simulink model "can8auto"  (R2018a)
settings: Solver=VariableStepAuto  StartTime=0.0  StopTime=5000  RelTol=1e-3
libraries: commcrc2 x20, simulink x20, simulink_extras x5, dspswit3 x5
(part 1 of 7)
settings Model: Creator=eugi  LastModifiedBy=Davide
settings DebuggingCC: UnderspecifiedInitializationDetection=Classic  LibraryContextMissingDiagnostic=warning
settings SFSimCC: SimUseLocalCustomCode=on
settings RTWCC: RTWUseLocalCustomCode=on

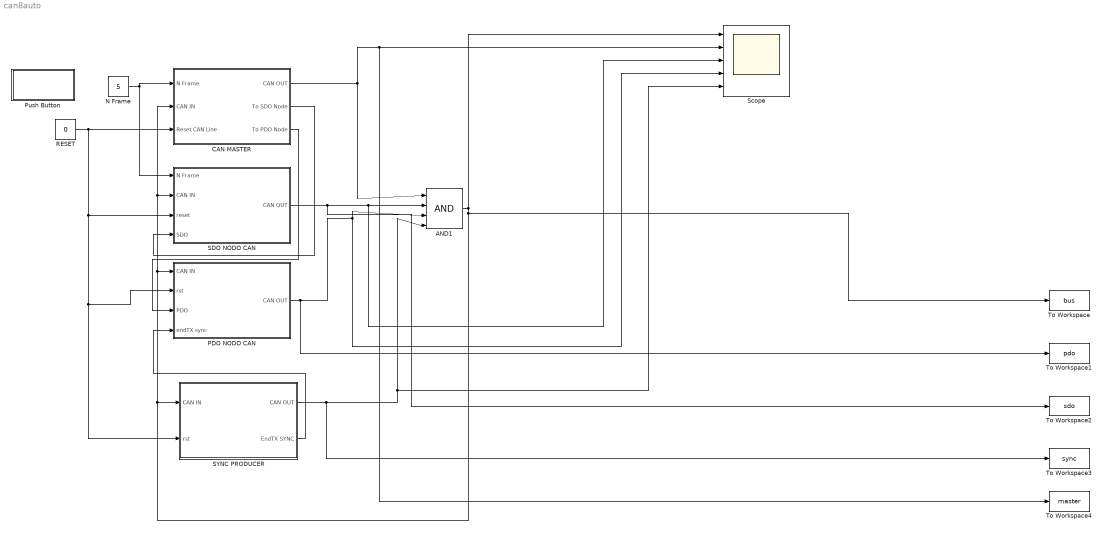
== system can8auto ==
  AND1 : Logic  Inputs=4  IconShape=distinctive  AllPortsSameDT=off  OutDataTypeStr=boolean
  CAN MASTER : Subsystem
  N Frame : Constant  Value=5
  "PDO NODO CAN " : Subsystem
  Push Button : Subsystem  DialogController=hmiCreateDDGDialog  IsWebBlock=on  mask(MWDashboardBlock){webBlockId=d599c260-cdec-44c3-9960-ce2c37887e91, webBlockType=pushbutton, ShowInLibBrowser=on, ShowInitialText=on, HMISrcModelName=can8auto}
      mask prompts: webBlockId "WebBlock Id"; webBlockType "WebBlock Type"; HMISrcModelName "Source Model"
      mask help: Set a value of a tunable parameter or variable by selecting and holding the button. When the push button is not selected, the value is set back to the default value.
      mask Help: helpview([docroot '/mapfiles/simulink.map'], 'hmi_pushbutton')
      mask Display:
      | if strcmp(get_param(bdroot(gcb),'BlockDiagramType'),'library')
      |  image([(matlabroot) '/toolbox/simulink/hmi/icons/PushButton.png'])
      | end
  RESET : Constant  Value=0
  SDO NODO CAN : Subsystem
  SYNC PRODUCER : Subsystem
  Scope : Scope  NumInputPorts=5
  To Workspace : ToWorkspace  VariableName=bus  SaveFormat=Timeseries  SampleTime=-1
  To Workspace1 : ToWorkspace  VariableName=pdo  SaveFormat=Timeseries  SampleTime=-1
  To Workspace2 : ToWorkspace  VariableName=sdo  SaveFormat=Timeseries  SampleTime=-1
  To Workspace3 : ToWorkspace  VariableName=sync  SaveFormat=Timeseries  SampleTime=-1
  To Workspace4 : ToWorkspace  VariableName=master  SaveFormat=Timeseries  SampleTime=-1
  wires:
  N Frame/1 -> SDO NODO CAN/1(N Frame), CAN MASTER/1(N Frame)
  RESET/1 -> CAN MASTER/3(Reset CAN Line), SDO NODO CAN/3(reset), "PDO NODO CAN "/2(rst), SYNC PRODUCER/2(rst)
  CAN MASTER/2(To SDO Node) -> SDO NODO CAN/4(SDO)
  CAN MASTER/3(To PDO Node) -> "PDO NODO CAN "/3(PDO)
  SYNC PRODUCER/2(EndTX SYNC) -> "PDO NODO CAN "/4(endTX sync)
  CAN MASTER/1(CAN OUT) -> AND1/1, To Workspace4/1, Scope/2
  SYNC PRODUCER/1(CAN OUT) -> To Workspace3/1, AND1/4, Scope/5
  SDO NODO CAN/1(CAN OUT) -> To Workspace2/1, Scope/3, AND1/2
  AND1/1 -> Scope/1, To Workspace/1, SYNC PRODUCER/1(CAN IN), SDO NODO CAN/2(CAN IN), CAN MASTER/2(CAN IN), "PDO NODO CAN "/1(CAN IN)
  "PDO NODO CAN "/1(CAN OUT) -> To Workspace1/1, Scope/4, AND1/3

== system can8auto/CAN MASTER ==
  N Frame : Inport
  CAN IN : Inport  Port=2
  Reset CAN Line : Inport  Port=3
  CAN NODE : Subsystem
  Chart : Stateflow chart  TreatAsAtomicUnit=on
  Clock : simulink_extras/Flip Flops/Clock  period=0.000001
  Constant : Constant
  Counter : dspswit3/Counter  Direction=Up  CountEvent=Rising edge  CounterSize=User defined  MaxCount=255  InitialCount=0  Output=Count and Hit  HitValue=32  ResetInput=on  SamplesPerFrame=1  Ts=1  CntDtype=double  HitDtype=Logical
  Counter1 : dspswit3/Counter  Direction=Up  CountEvent=Rising edge  CounterSize=User defined  MaxCount=255  InitialCount=0  Output=Count and Hit  HitValue=32  ResetInput=on  SamplesPerFrame=1  Ts=1  CntDtype=double  HitDtype=Logical
  Equal : RelationalOperator  Operator=~=  OutDataTypeStr=boolean  RndMeth=Simplest
  MATLAB Function : MATLAB Function  TreatAsAtomicUnit=on
  MATLAB Function1 : MATLAB Function  TreatAsAtomicUnit=on
  Master : Stateflow chart  TreatAsAtomicUnit=on
  Memory1 : Memory  InitialCondition=1
  Memory2 : Memory  InheritSampleTime=on
  Memory3 : Memory
  Sensing : Subsystem
  Sum : Sum  Inputs=|++
  XOR : Logic  Operator=XOR  IconShape=distinctive  AllPortsSameDT=off  OutDataTypeStr=boolean
  CAN OUT : Outport
  To SDO Node : Outport  Port=2
  To PDO Node : Outport  Port=3
  wires:
  Chart/1(state) -> Sensing/3(Enable CS), MATLAB Function/3(state)
  Clock/1 -> MATLAB Function/Trigger, Sensing/2(clock)
  Sensing/1(Free) -> Chart/1(Free)
  CAN IN/1 -> XOR/1, Sensing/1(BusState)
  XOR/1 -> Memory3/1
  CAN NODE/1(Frame Message) -> MATLAB Function/1(parallel)
  Memory1/1 -> MATLAB Function/2(current_index)
  MATLAB Function/2(next_index) -> Memory1/1
  MATLAB Function/1(serial) -> MATLAB Function1/1(u)
  MATLAB Function/3(endTX) -> Memory2/1
  MATLAB Function1/1(y) -> CAN OUT/1, XOR/2
  Memory3/1 -> Chart/2(Error)
  Memory2/1 -> Counter1/1, CAN NODE/1(End TX), Counter/1, Master/2(EndTX), Chart/4(EndTX)
  Master/3(sigOut) -> CAN NODE/2(TX Kind)
  Reset CAN Line/1 -> Counter/2, Master/1(rst)
  Master/1(SDO) -> To SDO Node/1
  Master/2(PDO) -> To PDO Node/1
  Counter/1 -> Master/3(totalTX)
  Counter1/1 -> Equal/2
  Equal/1 -> Chart/3(Frame)
  Constant/1 -> Sum/2
  N Frame/1 -> Sum/1
  Sum/1 -> Equal/1

== system can8auto/PDO NODO CAN  ==
  CAN IN : Inport
  rst : Inport  Port=2
  PDO : Inport  Port=3
  endTX sync : Inport  Port=4
  AND : Logic  IconShape=distinctive  AllPortsSameDT=off  OutDataTypeStr=boolean
  CAN NODE : Subsystem
  Chart : Stateflow chart  TreatAsAtomicUnit=on
  Clock : simulink_extras/Flip Flops/Clock  period=0.000001
  Counter of Sync Messages : Subsystem
  Delay : Delay  DelayLength=3
  Delay1 : Delay
  MATLAB Function : MATLAB Function  TreatAsAtomicUnit=on
  MATLAB Function1 : MATLAB Function  TreatAsAtomicUnit=on
  MATLAB Function2 : MATLAB Function  TreatAsAtomicUnit=on
  Memory1 : Memory  InitialCondition=1
  Memory2 : Memory  InheritSampleTime=on
  Memory3 : Memory
  NOT : Logic  Operator=NOT  IconShape=distinctive  AllPortsSameDT=off  OutDataTypeStr=boolean
  OR : Logic  Operator=OR  IconShape=distinctive  AllPortsSameDT=off  OutDataTypeStr=boolean
  Rate Transition : RateTransition
  Sensing : Subsystem
  SlavePDO : Stateflow chart  TreatAsAtomicUnit=on
  Start on push : Subsystem
  XOR : Logic  Operator=XOR  IconShape=distinctive  AllPortsSameDT=off  OutDataTypeStr=boolean
  CAN OUT : Outport
  wires:
  Chart/1(state) -> Sensing/3(Enable CS), MATLAB Function/3(state)
  Clock/1 -> AND/2, Start on push/1(New TX), MATLAB Function/Trigger, Sensing/2(clock)
  Sensing/1(Free) -> Chart/1(Free)
  CAN IN/1 -> XOR/1, Sensing/1(BusState)
  XOR/1 -> Memory3/1
  CAN NODE/1(Frame Message) -> MATLAB Function/1(parallel)
  Memory1/1 -> MATLAB Function/2(current_index)
  MATLAB Function/2(next_index) -> Memory1/1
  MATLAB Function/1(serial) -> MATLAB Function1/1(u)
  MATLAB Function/3(endTX) -> Memory2/1
  MATLAB Function1/1(y) -> CAN OUT/1, XOR/2
  Memory2/1 -> OR/2, Counter of Sync Messages/2(Down), SlavePDO/3(EndTX), Chart/4(EndTX)
  Memory3/1 -> Chart/2(Error)
  SlavePDO/1(mode) -> NOT/1, CAN NODE/2("Tx kind "), Chart/6(mode)
  rst/1 -> SlavePDO/1(rst)
  PDO/1 -> SlavePDO/2(PDO)
  endTX sync/1 -> Counter of Sync Messages/1(Up)
  Counter of Sync Messages/1(NFrame) -> Rate Transition/1
  Rate Transition/1 -> Chart/3(trigger)
  AND/1 -> OR/1
  NOT/1 -> AND/1
  Start on push/1(Out1) -> Delay/1
  Delay/1 -> Chart/5(NewTX)
  OR/1 -> Delay1/1
  Delay1/1 -> CAN NODE/1(Transmission Ready)

== system can8auto/Push Button ==

== system can8auto/SDO NODO CAN ==
  N Frame : Inport
  CAN IN : Inport  Port=2
  reset : Inport  Port=3
  SDO : Inport  Port=4
  CAN NODE : Subsystem
  Chart : Stateflow chart  TreatAsAtomicUnit=on
  Clock : simulink_extras/Flip Flops/Clock  period=0.000001
  Constant : Constant
  Counter : dspswit3/Counter  Direction=Up  CountEvent=Rising edge  CounterSize=User defined  MaxCount=255  InitialCount=0  Output=Count and Hit  HitValue=32  ResetInput=on  SamplesPerFrame=1  Ts=1  CntDtype=double  HitDtype=Logical
  Counter1 : dspswit3/Counter  Direction=Up  CountEvent=Rising edge  CounterSize=User defined  MaxCount=255  InitialCount=0  Output=Count and Hit  HitValue=32  ResetInput=on  SamplesPerFrame=1  Ts=1  CntDtype=double  HitDtype=Logical
  Equal : RelationalOperator  Operator=~=  OutDataTypeStr=boolean  RndMeth=Simplest
  MATLAB Function : MATLAB Function  TreatAsAtomicUnit=on
  MATLAB Function1 : MATLAB Function  TreatAsAtomicUnit=on
  Memory1 : Memory  InitialCondition=1
  Memory2 : Memory  InheritSampleTime=on
  Memory3 : Memory
  Sensing : Subsystem
  SlaveSDO : Stateflow chart  TreatAsAtomicUnit=on
  Sum : Sum  Inputs=|++
  XOR : Logic  Operator=XOR  IconShape=distinctive  AllPortsSameDT=off  OutDataTypeStr=boolean
  CAN OUT : Outport
  wires:
  Chart/1(state) -> Sensing/3(Enable CS), MATLAB Function/3(state)
  Clock/1 -> MATLAB Function/Trigger, Sensing/2(clock)
  Sensing/1(Free) -> Chart/1(Free)
  CAN IN/1 -> XOR/1, Sensing/1(BusState)
  XOR/1 -> Memory3/1
  CAN NODE/1(Frame Message) -> MATLAB Function/1(parallel)
  Memory1/1 -> MATLAB Function/2(current_index)
  MATLAB Function/2(next_index) -> Memory1/1
  MATLAB Function/1(serial) -> MATLAB Function1/1(u)
  MATLAB Function/3(endTX) -> Memory2/1
  MATLAB Function1/1(y) -> CAN OUT/1, XOR/2
  Memory3/1 -> Chart/2(Error)
  reset/1 -> Counter/2, SlaveSDO/1(rst)
  SDO/1 -> SlaveSDO/2(SDO)
  SlaveSDO/1(mode) -> CAN NODE/2(Frame kind)
  Counter/1 -> SlaveSDO/3(TotTX)
  Equal/1 -> Chart/3(Frame)
  Sum/1 -> Equal/1
  N Frame/1 -> Sum/1
  Counter1/1 -> Equal/2
  Constant/1 -> Sum/2
  Memory2/1 -> Counter1/1, Counter/1, SlaveSDO/4(EndTX), CAN NODE/1(End TX), Chart/4(EndTX)

== system can8auto/SYNC PRODUCER ==
  CAN IN : Inport
  rst : Inport  Port=2
  AND : Logic  Inputs=3  IconShape=distinctive  AllPortsSameDT=off  OutDataTypeStr=boolean
  CAN NODE : Subsystem
  Chart : Stateflow chart  TreatAsAtomicUnit=on
  Chart1 : Stateflow chart  TreatAsAtomicUnit=on
  Clock : simulink_extras/Flip Flops/Clock  period=0.000001
  Clock1 : simulink_extras/Flip Flops/Clock  period=0.000002
  Counter1 : dspswit3/Counter  Direction=Up  CountEvent=Rising edge  CounterSize=User defined  MaxCount=256  InitialCount=0  Output=Count and Hit  HitValue=256  ResetInput=on  SamplesPerFrame=1  Ts=1  CntDtype=double  HitDtype=Logical
  Delay : Delay  DelayLength=3
  Display2 : Display
  MATLAB Function : MATLAB Function  TreatAsAtomicUnit=on
  Memory : Memory
  Memory1 : Memory  InitialCondition=1
  Memory2 : Memory  InheritSampleTime=on
  Memory3 : Memory
  Memory4 : Memory  InheritSampleTime=on
  NOT : Logic  Operator=NOT  IconShape=distinctive  AllPortsSameDT=off  OutDataTypeStr=boolean
  OR : Logic  Operator=OR  IconShape=distinctive  AllPortsSameDT=off  OutDataTypeStr=boolean
  P/S converter : MATLAB Function  TreatAsAtomicUnit=on
  Rate Transition : RateTransition
  Sensing : Subsystem
  Start on push : Subsystem
  XOR : Logic  Operator=XOR  IconShape=distinctive  AllPortsSameDT=off  OutDataTypeStr=boolean
  double to boolean : MATLAB Function  TreatAsAtomicUnit=on
  CAN OUT : Outport
  EndTX SYNC : Outport  Port=2
  wires:
  Chart/1(state) -> Sensing/3(Enable CS), Memory4/1, P/S converter/3(state)
  Sensing/1(Free) -> Chart/1(Free)
  CAN IN/1 -> XOR/1, Sensing/1(BusState)
  XOR/1 -> Memory3/1
  CAN NODE/1(Frame Message) -> P/S converter/1(parallel)
  Memory1/1 -> P/S converter/2(current_index)
  P/S converter/2(next_index) -> Memory1/1
  P/S converter/1(serial) -> double to boolean/1(u)
  P/S converter/3(endTX) -> Memory2/1
  double to boolean/1(y) -> CAN OUT/1, XOR/2
  Memory2/1 -> OR/2, Chart1/1(EndTX), EndTX SYNC/1, Chart/3(EndTX)
  Memory3/1 -> Chart/2(Error)
  rst/1 -> Chart1/2(rst), OR/1
  Chart1/1(mode) -> Chart/6(mode), MATLAB Function/1(u), CAN NODE/2(tx kind)
  Clock1/1 -> AND/1
  AND/1 -> Counter1/1
  Memory/1 -> Rate Transition/1
  Rate Transition/1 -> AND/2
  Counter1/1 -> Display2/1
  Clock/1 -> Start on push/1(New TX), CAN NODE/1(Transmission Ready), P/S converter/Trigger, Sensing/2(clock)
  Start on push/1(Out1) -> Delay/1
  MATLAB Function/1(y) -> Memory/1
  Counter1/2 -> Chart/5(tempo)
  NOT/1 -> AND/3
  Memory4/1 -> NOT/1
  OR/1 -> Counter1/2
  Delay/1 -> Chart/4(enableTX)

== system can8auto/CAN MASTER/CAN NODE ==
  note: DA INSERIRE L'ID DEL NODO
      | (Node ID) & L'INDIRIZZO
      | RICEVITORE DI UN NMT NODE
      | (Address Node)
  note: TRANSMISSION TRIGGER
  note: MESSAGE CONIG
  End TX : Inport
  TX Kind : Inport  Port=2
  "Address Node " : Constant  Value=[0,0,0,0,0,0,0,0,0,0,0]  VectorParams1D=off
  Bootup Frame generator : Subsystem
  Complex to Real-Imag : ComplexToRealImag  Output=Real
  Frame MUX : Subsystem
  Length : Constant  Value=4  VectorParams1D=off
  Mode : Constant  VectorParams1D=off
  NMT Frame generator : Subsystem
  Node ID : Constant  Value=[0,0,1,0,0,0,0,1,1,1,1]  VectorParams1D=off
  PDO Frame Generator : Subsystem
  Radio Button : RadioButtonGroup  WebBlockId=15712  LabelPosition=Hide  SelectedLabel=Bootup Message  ButtonGroupName=Message
      settings: Values={{'Bootup Message', 'NMT Message', 'SDO Message', 'PDO Message', 'SYNC Message'}, [0 1 2 3 4]}
  Radio Button1 : RadioButtonGroup  WebBlockId=15713  LabelPosition=Hide  SelectedLabel=WriteClent  ButtonGroupName=SDO request
      settings: Values={{'ReadClient', 'WriteClent', 'ReadServer', 'WriteServer'}, [0 1 2 3]}
  Radio Button2 : RadioButtonGroup  WebBlockId=15714  LabelPosition=Hide  SelectedLabel=4 Byte  ButtonGroupName=PDO Length
      settings: Values={{'2 Byte', '4 Byte', '8 Byte'}, [2 4 8]}
  SDO Frame generator : Subsystem
  SYNC Frame Generator : Subsystem
  Triggered Subsystem1 : Subsystem  TreatAsAtomicUnit=on
  Frame Message : Outport
  wires:
  Complex to Real-Imag/1 -> Frame Message/1
  Frame MUX/1(Frame to Send) -> Triggered Subsystem1/1(In1)
  "Address Node "/1 -> NMT Frame generator/1(Address node)
  TX Kind/1 -> Frame MUX/1(Frame Kind)
  NMT Frame generator/2(" Size") -> Frame MUX/5(Size NMT)
  SYNC Frame Generator/2(" Size") -> Frame MUX/11(Size SYNC)
  Mode/1 -> SDO Frame generator/2(Mode)
  Length/1 -> PDO Frame Generator/2(Data Length)
  Bootup Frame generator/2(" Size") -> Frame MUX/3(Size Bootload)
  SDO Frame generator/2(" Size") -> Frame MUX/7(Size SDO)
  Node ID/1 -> Bootup Frame generator/1(ID of the Node), PDO Frame Generator/1(CAN ID), SDO Frame generator/1(CAN ID of the Node)
  NMT Frame generator/1(NMT Frame) -> Frame MUX/4(NMT Frame)
  PDO Frame Generator/2(" Size") -> Frame MUX/9(Size PDO)
  SDO Frame generator/1(SDO Frame) -> Frame MUX/6(SDO Frame)
  SYNC Frame Generator/1(SYNC Frame) -> Frame MUX/10(SYNC Frame)
  Bootup Frame generator/1(Bootload Frame) -> Frame MUX/2(Bootload Frame)
  PDO Frame Generator/1(PDO Frame) -> Frame MUX/8(PDO Frame)
  Triggered Subsystem1/1(Out1) -> Complex to Real-Imag/1
  End TX/1 -> Triggered Subsystem1/Trigger

== system can8auto/CAN MASTER/Sensing ==
  BusState : Inport
  clock : Inport  Port=2
  Enable CS : Inport  Port=3
  AND : Logic  IconShape=distinctive  AllPortsSameDT=off  OutDataTypeStr=boolean
  Data Store Memory : DataStoreMemory  ReadBeforeWriteMsg=warning  WriteAfterWriteMsg=warning  WriteAfterReadMsg=warning  ShowAdditionalParam=off
  Data Store Read : DataStoreRead
  Data Store Write : DataStoreWrite
  MATLAB Function : MATLAB Function  TreatAsAtomicUnit=on
  Memory : Memory
  NOT : Logic  Operator=NOT  IconShape=distinctive  AllPortsSameDT=off  OutDataTypeStr=boolean
  Free : Outport
  wires:
  Memory/1 -> Free/1
  Enable CS/1 -> AND/1
  AND/1 -> NOT/1
  clock/1 -> AND/2
  NOT/1 -> MATLAB Function/Trigger, MATLAB Function/2(clock)
  MATLAB Function/2(count) -> Data Store Write/1
  Data Store Read/1 -> MATLAB Function/3("count ")
  MATLAB Function/1(free) -> Memory/1
  BusState/1 -> MATLAB Function/1(BusState)

== system can8auto/PDO NODO CAN /CAN NODE ==
  note: DA INSERIRE L'ID DEL NODO
      | (Node ID) & L'INDIRIZZO
      | RICEVITORE DI UN NMT NODE
      | (Address Node)
  note: TRANSMISSION TRIGGER
  note: MESSAGE CONIG
  Transmission Ready : Inport
  "Tx kind " : Inport  Port=2
  "Address Node " : Constant  Value=[0,0,0,0,0,0,0,0,0,0,0]  VectorParams1D=off
  Bootup Frame generator : Subsystem
  Complex to Real-Imag : ComplexToRealImag  Output=Real
  Frame MUX : Subsystem
  Length : Constant  Value=4  VectorParams1D=off
  Mode : Constant  VectorParams1D=off
  NMT Frame generator : Subsystem
  Node ID : Constant  Value=[0,0,1,1,0,0,0,0,1,0,1]  VectorParams1D=off
  PDO Frame Generator : Subsystem
  Radio Button : RadioButtonGroup  WebBlockId=13844  LabelPosition=Hide  SelectedLabel=Bootup Message  ButtonGroupName=Message
      settings: Values={{'Bootup Message', 'NMT Message', 'SDO Message', 'PDO Message', 'SYNC Message'}, [0 1 2 3 4]}
  Radio Button1 : RadioButtonGroup  WebBlockId=13845  LabelPosition=Hide  SelectedLabel=WriteClent  ButtonGroupName=SDO request
      settings: Values={{'ReadClient', 'WriteClent', 'ReadServer', 'WriteServer'}, [0 1 2 3]}
  Radio Button2 : RadioButtonGroup  WebBlockId=13846  LabelPosition=Hide  SelectedLabel=4 Byte  ButtonGroupName=PDO Length
      settings: Values={{'2 Byte', '4 Byte', '8 Byte'}, [2 4 8]}
  SDO Frame generator : Subsystem
  SYNC Frame Generator : Subsystem
  Triggered Subsystem1 : Subsystem  TreatAsAtomicUnit=on
  Frame Message : Outport
  wires:
  Transmission Ready/1 -> Triggered Subsystem1/Trigger
  Complex to Real-Imag/1 -> Frame Message/1
  Frame MUX/1(Frame to Send) -> Triggered Subsystem1/1(In1)
  "Address Node "/1 -> NMT Frame generator/1(Address node)
  "Tx kind "/1 -> Frame MUX/1(Frame Kind)
  NMT Frame generator/2(" Size") -> Frame MUX/5(Size NMT)
  SYNC Frame Generator/2(" Size") -> Frame MUX/11(Size SYNC)
  Mode/1 -> SDO Frame generator/2(Mode)
  Length/1 -> PDO Frame Generator/2(Data Length)
  Bootup Frame generator/2(" Size") -> Frame MUX/3(Size Bootload)
  SDO Frame generator/2(" Size") -> Frame MUX/7(Size SDO)
  Node ID/1 -> Bootup Frame generator/1(ID of the Node), PDO Frame Generator/1(CAN ID), SDO Frame generator/1(CAN ID of the Node)
  NMT Frame generator/1(NMT Frame) -> Frame MUX/4(NMT Frame)
  PDO Frame Generator/2(" Size") -> Frame MUX/9(Size PDO)
  SDO Frame generator/1(SDO Frame) -> Frame MUX/6(SDO Frame)
  SYNC Frame Generator/1(SYNC Frame) -> Frame MUX/10(SYNC Frame)
  Bootup Frame generator/1(Bootload Frame) -> Frame MUX/2(Bootload Frame)
  PDO Frame Generator/1(PDO Frame) -> Frame MUX/8(PDO Frame)
  Triggered Subsystem1/1(Out1) -> Complex to Real-Imag/1

== system can8auto/PDO NODO CAN /Counter of Sync Messages ==
  Up : Inport
  Down : Inport  Port=2
  ADDER : MATLAB Function  TreatAsAtomicUnit=on
  Memory : Memory
  OR : Logic  Operator=OR  IconShape=distinctive  AllPortsSameDT=off  OutDataTypeStr=boolean
  NFrame : Outport
  wires:
  Up/1 -> ADDER/1(up), OR/2
  Memory/1 -> ADDER/3(counter), NFrame/1
  Down/1 -> ADDER/2(down), OR/1
  OR/1 -> ADDER/Trigger
  ADDER/1(val) -> Memory/1

== system can8auto/PDO NODO CAN /Sensing ==
  BusState : Inport
  clock : Inport  Port=2
  Enable CS : Inport  Port=3
  AND : Logic  IconShape=distinctive  AllPortsSameDT=off  OutDataTypeStr=boolean
  Data Store Memory : DataStoreMemory  ReadBeforeWriteMsg=warning  WriteAfterWriteMsg=warning  WriteAfterReadMsg=warning  ShowAdditionalParam=off
  Data Store Read : DataStoreRead
  Data Store Write : DataStoreWrite
  MATLAB Function : MATLAB Function  TreatAsAtomicUnit=on
  Memory : Memory
  NOT : Logic  Operator=NOT  IconShape=distinctive  AllPortsSameDT=off  OutDataTypeStr=boolean
  Free : Outport
  wires:
  Memory/1 -> Free/1
  Enable CS/1 -> AND/1
  AND/1 -> NOT/1
  clock/1 -> AND/2
  NOT/1 -> MATLAB Function/Trigger, MATLAB Function/2(clock)
  MATLAB Function/2(count) -> Data Store Write/1
  Data Store Read/1 -> MATLAB Function/3("count ")
  MATLAB Function/1(free) -> Memory/1
  BusState/1 -> MATLAB Function/1(BusState)

== system can8auto/PDO NODO CAN /Start on push ==
  New TX : Inport
  Constant : Constant
  Start on push : Subsystem  TreatAsAtomicUnit=on
  Out1 : Outport
  wires:
  Start on push/1(Out1) -> Out1/1
  New TX/1 -> Start on push/Trigger
  Constant/1 -> Start on push/1(In1)

== system can8auto/SDO NODO CAN/CAN NODE ==
  note: DA INSERIRE L'ID DEL NODO
      | (Node ID) & L'INDIRIZZO
      | RICEVITORE DI UN NMT NODE
      | (Address Node)
  note: TRANSMISSION TRIGGER
  note: MESSAGE CONIG
  End TX : Inport
  Frame kind : Inport  Port=2
  "Address Node " : Constant  Value=[0,0,0,0,0,0,0,0,0,0,0]  VectorParams1D=off
  Bootup Frame generator : Subsystem
  Complex to Real-Imag : ComplexToRealImag  Output=Real
  Frame MUX : Subsystem
  Length : Constant  Value=4  VectorParams1D=off
  Mode : Constant  VectorParams1D=off
  NMT Frame generator : Subsystem
  Node ID : Constant  Value=[0,0,1,1,0,0,1,0,1,0,1]  VectorParams1D=off
  PDO Frame Generator : Subsystem
  Radio Button : RadioButtonGroup  WebBlockId=16646  LabelPosition=Hide  SelectedLabel=Bootup Message  ButtonGroupName=Message
      settings: Values={{'Bootup Message', 'NMT Message', 'SDO Message', 'PDO Message', 'SYNC Message'}, [0 1 2 3 4]}
  Radio Button1 : RadioButtonGroup  WebBlockId=16647  LabelPosition=Hide  SelectedLabel=WriteClent  ButtonGroupName=SDO request
      settings: Values={{'ReadClient', 'WriteClent', 'ReadServer', 'WriteServer'}, [0 1 2 3]}
  Radio Button2 : RadioButtonGroup  WebBlockId=16648  LabelPosition=Hide  SelectedLabel=4 Byte  ButtonGroupName=PDO Length
      settings: Values={{'2 Byte', '4 Byte', '8 Byte'}, [2 4 8]}
  SDO Frame generator : Subsystem
  SYNC Frame Generator : Subsystem
  Triggered Subsystem1 : Subsystem  TreatAsAtomicUnit=on
  Frame Message : Outport
  wires:
  Complex to Real-Imag/1 -> Frame Message/1
  Frame MUX/1(Frame to Send) -> Triggered Subsystem1/1(In1)
  "Address Node "/1 -> NMT Frame generator/1(Address node)
  Frame kind/1 -> Frame MUX/1(Frame Kind)
  NMT Frame generator/2(" Size") -> Frame MUX/5(Size NMT)
  SYNC Frame Generator/2(" Size") -> Frame MUX/11(Size SYNC)
  Mode/1 -> SDO Frame generator/2(Mode)
  Length/1 -> PDO Frame Generator/2(Data Length)
  Bootup Frame generator/2(" Size") -> Frame MUX/3(Size Bootload)
  SDO Frame generator/2(" Size") -> Frame MUX/7(Size SDO)
  Node ID/1 -> Bootup Frame generator/1(ID of the Node), PDO Frame Generator/1(CAN ID), SDO Frame generator/1(CAN ID of the Node)
  NMT Frame generator/1(NMT Frame) -> Frame MUX/4(NMT Frame)
  PDO Frame Generator/2(" Size") -> Frame MUX/9(Size PDO)
  SDO Frame generator/1(SDO Frame) -> Frame MUX/6(SDO Frame)
  SYNC Frame Generator/1(SYNC Frame) -> Frame MUX/10(SYNC Frame)
  Bootup Frame generator/1(Bootload Frame) -> Frame MUX/2(Bootload Frame)
  PDO Frame Generator/1(PDO Frame) -> Frame MUX/8(PDO Frame)
  Triggered Subsystem1/1(Out1) -> Complex to Real-Imag/1
  End TX/1 -> Triggered Subsystem1/Trigger

== system can8auto/SDO NODO CAN/Sensing ==
  BusState : Inport
  clock : Inport  Port=2
  Enable CS : Inport  Port=3
  AND : Logic  IconShape=distinctive  AllPortsSameDT=off  OutDataTypeStr=boolean
  Data Store Memory : DataStoreMemory  ReadBeforeWriteMsg=warning  WriteAfterWriteMsg=warning  WriteAfterReadMsg=warning  ShowAdditionalParam=off
  Data Store Read : DataStoreRead
  Data Store Write : DataStoreWrite
  MATLAB Function : MATLAB Function  TreatAsAtomicUnit=on
  Memory : Memory
  NOT : Logic  Operator=NOT  IconShape=distinctive  AllPortsSameDT=off  OutDataTypeStr=boolean
  Free : Outport
  wires:
  Memory/1 -> Free/1
  Enable CS/1 -> AND/1
  AND/1 -> NOT/1
  clock/1 -> AND/2
  NOT/1 -> MATLAB Function/Trigger, MATLAB Function/2(clock)
  MATLAB Function/2(count) -> Data Store Write/1
  Data Store Read/1 -> MATLAB Function/3("count ")
  MATLAB Function/1(free) -> Memory/1
  BusState/1 -> MATLAB Function/1(BusState)

== system can8auto/SYNC PRODUCER/CAN NODE ==
  note: DA INSERIRE L'ID DEL NODO
      | (Node ID) & L'INDIRIZZO
      | RICEVITORE DI UN NMT NODE
      | (Address Node)
  note: TRANSMISSION TRIGGER
  note: MESSAGE CONIG
  Transmission Ready : Inport
  tx kind : Inport  Port=2
  "Address Node " : Constant  Value=[0,0,0,0,0,0,0,0,0,0,0]  VectorParams1D=off
  Bootup Frame generator : Subsystem
  Complex to Real-Imag : ComplexToRealImag  Output=Real
  Frame MUX : Subsystem
  Length : Constant  Value=4  VectorParams1D=off
  Mode : Constant  VectorParams1D=off
  NMT Frame generator : Subsystem
  Node ID : Constant  Value=[0,0,1,0,0,0,0,1,1,0,1]  VectorParams1D=off
  PDO Frame Generator : Subsystem
  Radio Button1 : RadioButtonGroup  WebBlockId=17625  LabelPosition=Hide  SelectedLabel=WriteClent  ButtonGroupName=SDO request
      settings: Values={{'ReadClient', 'WriteClent', 'ReadServer', 'WriteServer'}, [0 1 2 3]}
  Radio Button2 : RadioButtonGroup  WebBlockId=17626  LabelPosition=Hide  SelectedLabel=4 Byte  ButtonGroupName=PDO Length
      settings: Values={{'2 Byte', '4 Byte', '8 Byte'}, [2 4 8]}
  SDO Frame generator : Subsystem
  SYNC Frame Generator : Subsystem
  Triggered Subsystem1 : Subsystem  TreatAsAtomicUnit=on
  Frame Message : Outport
  wires:
  Transmission Ready/1 -> Triggered Subsystem1/Trigger
  Complex to Real-Imag/1 -> Frame Message/1
  Frame MUX/1(Frame to Send) -> Triggered Subsystem1/1(In1)
  "Address Node "/1 -> NMT Frame generator/1(Address node)
  tx kind/1 -> Frame MUX/1(Frame Kind)
  NMT Frame generator/2(" Size") -> Frame MUX/5(Size NMT)
  SYNC Frame Generator/2(" Size") -> Frame MUX/11(Size SYNC)
  Mode/1 -> SDO Frame generator/2(Mode)
  Length/1 -> PDO Frame Generator/2(Data Length)
  Bootup Frame generator/2(" Size") -> Frame MUX/3(Size Bootload)
  SDO Frame generator/2(" Size") -> Frame MUX/7(Size SDO)
  Node ID/1 -> Bootup Frame generator/1(ID of the Node), PDO Frame Generator/1(CAN ID), SDO Frame generator/1(CAN ID of the Node)
  NMT Frame generator/1(NMT Frame) -> Frame MUX/4(NMT Frame)
  PDO Frame Generator/2(" Size") -> Frame MUX/9(Size PDO)
  SDO Frame generator/1(SDO Frame) -> Frame MUX/6(SDO Frame)
  SYNC Frame Generator/1(SYNC Frame) -> Frame MUX/10(SYNC Frame)
  Bootup Frame generator/1(Bootload Frame) -> Frame MUX/2(Bootload Frame)
  PDO Frame Generator/1(PDO Frame) -> Frame MUX/8(PDO Frame)
  Triggered Subsystem1/1(Out1) -> Complex to Real-Imag/1

== system can8auto/SYNC PRODUCER/Sensing ==
  BusState : Inport
  clock : Inport  Port=2
  Enable CS : Inport  Port=3
  AND : Logic  IconShape=distinctive  AllPortsSameDT=off  OutDataTypeStr=boolean
  Data Store Memory : DataStoreMemory  ReadBeforeWriteMsg=warning  WriteAfterWriteMsg=warning  WriteAfterReadMsg=warning  ShowAdditionalParam=off
  Data Store Read : DataStoreRead
  Data Store Write : DataStoreWrite
  MATLAB Function : MATLAB Function  TreatAsAtomicUnit=on
  Memory : Memory
  NOT : Logic  Operator=NOT  IconShape=distinctive  AllPortsSameDT=off  OutDataTypeStr=boolean
  Free : Outport
  wires:
  Memory/1 -> Free/1
  Enable CS/1 -> AND/1
  AND/1 -> NOT/1
  clock/1 -> AND/2
  NOT/1 -> MATLAB Function/Trigger, MATLAB Function/2(clock)
  MATLAB Function/2(count) -> Data Store Write/1
  Data Store Read/1 -> MATLAB Function/3("count ")
  MATLAB Function/1(free) -> Memory/1
  BusState/1 -> MATLAB Function/1(BusState)

== system can8auto/SYNC PRODUCER/Start on push ==
  New TX : Inport
  Constant : Constant
  Start on push : Subsystem  TreatAsAtomicUnit=on
  Out1 : Outport
  wires:
  Start on push/1(Out1) -> Out1/1
  New TX/1 -> Start on push/Trigger
  Constant/1 -> Start on push/1(In1)

== system can8auto/CAN MASTER/CAN NODE/Bootup Frame generator ==
  note: CAN ID / COB ID
  ID of the Node : Inport
  11-bit Adder : Subsystem
  700h : Constant  Value=[1,1,1,0,0,0,0,0,0,0,0]  VectorParams1D=off
  ACK : Constant  Value=[1,1]  VectorParams1D=off
  BitStuffing : Subsystem
  CRC delimiter : Constant  VectorParams1D=off
  Control : Constant  Value=[0,0,0,0,0,1]  VectorParams1D=off
  "Data (Bootup State) " : Constant  Value=[0,0,0,0,0,0,0,0]'  VectorParams1D=off
  EOF : Constant  Value=[1,1,1,1,1,1,0]  VectorParams1D=off
  General CRC Generator : commcrc2/General CRC Generator  genPoly='z^15 + z^14 + z^10 + z^8 + z^7 + z^4 + z^3 + 1'  iniStates=0  directMethod=off  reflectInputBytes=off  reflectChecksums=off  finalXOR=0  numChecksums=1
      settings: SourceProductName=Communications Toolbox  SourceProductBaseCode=CM
  Mux : Mux  Inputs=3
  Mux1 : Mux  Inputs=2
  Mux2 : Mux  Inputs=3
  Mux3 : Mux  Inputs=3
  RTR : Constant  Value=0  VectorParams1D=off
  SOF : Constant  Value=0  VectorParams1D=off
  Transpose : Math  Operator=transpose  SaturateOnIntegerOverflow=on
  Width : Width
  Bootload Frame : Outport
  " Size" : Outport  Port=2
  wires:
  Mux1/1 -> Mux3/1
  Mux2/1 -> Mux3/3
  BitStuffing/1(Out1) -> Mux3/2
  Mux3/1 -> Bootload Frame/1, Width/1
  Transpose/1 -> Mux/3
  RTR/1 -> Mux/1
  EOF/1 -> Mux2/3
  ACK/1 -> Mux2/2
  CRC delimiter/1 -> Mux2/1
  SOF/1 -> Mux1/1
  11-bit Adder/1(Out1) -> Mux1/2
  Width/1 -> " Size"/1
  ID of the Node/1 -> 11-bit Adder/2(In2)
  700h/1 -> 11-bit Adder/1(In1)
  Control/1 -> Mux/2
  "Data (Bootup State) "/1 -> General CRC Generator/1
  General CRC Generator/1 -> Transpose/1
  Mux/1 -> BitStuffing/1(In1)

== system can8auto/CAN MASTER/CAN NODE/Frame MUX ==
  Frame Kind : Inport
  Bootload Frame : Inport  Port=2
  Size Bootload : Inport  Port=3
  NMT Frame : Inport  Port=4
  Size NMT : Inport  Port=5
  SDO Frame : Inport  Port=6
  Size SDO : Inport  Port=7
  PDO Frame : Inport  Port=8
  Size PDO : Inport  Port=9
  SYNC Frame : Inport  Port=10
  Size SYNC : Inport  Port=11
  MATLAB Function2 : MATLAB Function  TreatAsAtomicUnit=on
  Vector Concatenate : Concatenate  NumInputs=5
  Vector Concatenate1 : Concatenate  NumInputs=5
  Frame to Send : Outport
  wires:
  Vector Concatenate1/1 -> MATLAB Function2/3(size)
  SYNC Frame/1 -> Vector Concatenate/5
  Size NMT/1 -> Vector Concatenate1/2
  Size SDO/1 -> Vector Concatenate1/3
  Size Bootload/1 -> Vector Concatenate1/1
  Size SYNC/1 -> Vector Concatenate1/5
  Vector Concatenate/1 -> MATLAB Function2/2(u1)
  SDO Frame/1 -> Vector Concatenate/3
  MATLAB Function2/1(result) -> Frame to Send/1
  Bootload Frame/1 -> Vector Concatenate/1
  PDO Frame/1 -> Vector Concatenate/4
  Frame Kind/1 -> MATLAB Function2/1(mode)
  NMT Frame/1 -> Vector Concatenate/2
  Size PDO/1 -> Vector Concatenate1/4

== system can8auto/CAN MASTER/CAN NODE/NMT Frame generator ==
  note: DATA FIELD
  Address node : Inport
  11-bit Adder : Subsystem
  ACK : Constant  Value=[1,1]  VectorParams1D=off
  BitStuffing : Subsystem
  COB ID : Constant  Value=[0,0,0,0,0,0,0,0,0,0,0]  VectorParams1D=off
  CRC delimiter : Constant  VectorParams1D=off
  Control : Constant  Value=[0,0,0,0,1,0]  VectorParams1D=off
  DATA (part1) : Constant  Value=[0,0,0,0,0]  VectorParams1D=off
  "Data " : Constant  Value=[0,0,1,0,0,0,0,0,0,0,0]  VectorParams1D=off
  EOF : Constant  Value=[1,1,1,1,1,1,0]  VectorParams1D=off
  General CRC Generator : commcrc2/General CRC Generator  genPoly='z^15 + z^14 + z^10 + z^8 + z^7 + z^4 + z^3 + 1'  iniStates=0  directMethod=off  reflectInputBytes=off  reflectChecksums=off  finalXOR=0  numChecksums=1
      settings: SourceProductName=Communications Toolbox  SourceProductBaseCode=CM
  Mux : Mux  Inputs=3
  Mux1 : Mux  Inputs=2
  Mux2 : Mux  Inputs=2
  Mux3 : Mux  Inputs=3
  Mux4 : Mux  Inputs=3
  RTR : Constant  Value=0  VectorParams1D=off
  SOF : Constant  Value=0  VectorParams1D=off
  Transpose : Math  Operator=transpose  SaturateOnIntegerOverflow=on
  Transpose1 : Math  Operator=transpose  SaturateOnIntegerOverflow=on
  Width : Width
  NMT Frame : Outport
  " Size" : Outport  Port=2
  wires:
  Mux4/1 -> Width/1, NMT Frame/1
  Mux3/1 -> Mux4/3
  Mux2/1 -> Mux4/1
  BitStuffing/1(Out1) -> Mux4/2
  Mux/1 -> BitStuffing/1(In1)
  RTR/1 -> Mux/1
  CRC delimiter/1 -> Mux3/1
  ACK/1 -> Mux3/2
  EOF/1 -> Mux3/3
  SOF/1 -> Mux2/1
  COB ID/1 -> Mux2/2
  Width/1 -> " Size"/1
  Transpose1/1 -> General CRC Generator/1
  Mux1/1 -> Transpose1/1
  11-bit Adder/1(Out1) -> Mux1/2
  DATA (part1)/1 -> Mux1/1
  "Data "/1 -> 11-bit Adder/1(In1)
  Address node/1 -> 11-bit Adder/2(In2)
  Transpose/1 -> Mux/3
  Control/1 -> Mux/2
  General CRC Generator/1 -> Transpose/1

== system can8auto/CAN MASTER/CAN NODE/PDO Frame Generator ==
  note: PDO DATA field
  note: CONTROL field
  CAN ID : Inport
  Data Length : Inport  Port=2
  " default = 8" : SwitchCase  CaseConditions={2,4}
  2 byte : Constant  Value=[0,0,0,0,1,0]  VectorParams1D=off
  4 byte : Constant  Value=[0,0,0,1,0,0]  VectorParams1D=off
  8 byte : Constant  Value=[0,0,1,0,0,0]  VectorParams1D=off
  ACK : Constant  Value=[1,1]  VectorParams1D=off
  CRC delimiter : Constant  VectorParams1D=off
  EOF : Constant  Value=[1,1,1,1,1,1,0]  VectorParams1D=off
  Floor1 : Rounding  Operator=round
  General CRC Generator : commcrc2/General CRC Generator  genPoly='z^15 + z^14 + z^10 + z^8 + z^7 + z^4 + z^3 + 1'  iniStates=0  directMethod=off  reflectInputBytes=off  reflectChecksums=off  finalXOR=0  numChecksums=1
      settings: SourceProductName=Communications Toolbox  SourceProductBaseCode=CM
  Merge1 : Merge  Inputs=3
  RTR : Constant  Value=0  VectorParams1D=off
  SOF : Constant  Value=0  VectorParams1D=off
  Subsystem : Subsystem
  Switch Case Action Subsystem : Subsystem  TreatAsAtomicUnit=on
  Switch Case Action Subsystem1 : Subsystem  TreatAsAtomicUnit=on
  Switch Case Action Subsystem2 : Subsystem  TreatAsAtomicUnit=on
  Tapped Delay : simulink/Discrete/Tapped Delay  vinit=0  samptime=-1  NumDelays=8*8  DelayOrder=Oldest  includeCurrent=off
  Uniform Random for Bit : UniformRandomNumber  Minimum=0  SampleTime=0.01
  Vector Concatenate1 : Concatenate  NumInputs=8
  Width : Width
  PDO Frame : Outport
  " Size" : Outport  Port=2
  wires:
  Vector Concatenate1/1 -> PDO Frame/1, Width/1
  Width/1 -> " Size"/1
  ACK/1 -> Vector Concatenate1/7
  EOF/1 -> Vector Concatenate1/8
  General CRC Generator/1 -> Vector Concatenate1/5
  Switch Case Action Subsystem1/1(Out1) -> Merge1/2
  2 byte/1 -> Switch Case Action Subsystem/1(In1)
  Tapped Delay/1 -> Subsystem/1(Random Bits)
  RTR/1 -> Vector Concatenate1/3
  Uniform Random for Bit/1 -> Floor1/1
  " default = 8"/3 -> Switch Case Action Subsystem2/Action
  Floor1/1 -> Tapped Delay/1
  SOF/1 -> Vector Concatenate1/1
  Data Length/1 -> " default = 8"/1, Subsystem/2(Length of Field)
  4 byte/1 -> Switch Case Action Subsystem1/1(In1)
  Subsystem/1(Generated Field) -> General CRC Generator/1
  " default = 8"/1 -> Switch Case Action Subsystem/Action
  CRC delimiter/1 -> Vector Concatenate1/6
  Merge1/1 -> Vector Concatenate1/4
  " default = 8"/2 -> Switch Case Action Subsystem1/Action
  8 byte/1 -> Switch Case Action Subsystem2/1(In1)
  CAN ID/1 -> Vector Concatenate1/2
  Switch Case Action Subsystem2/1(Out1) -> Merge1/3
  Switch Case Action Subsystem/1(Out1) -> Merge1/1

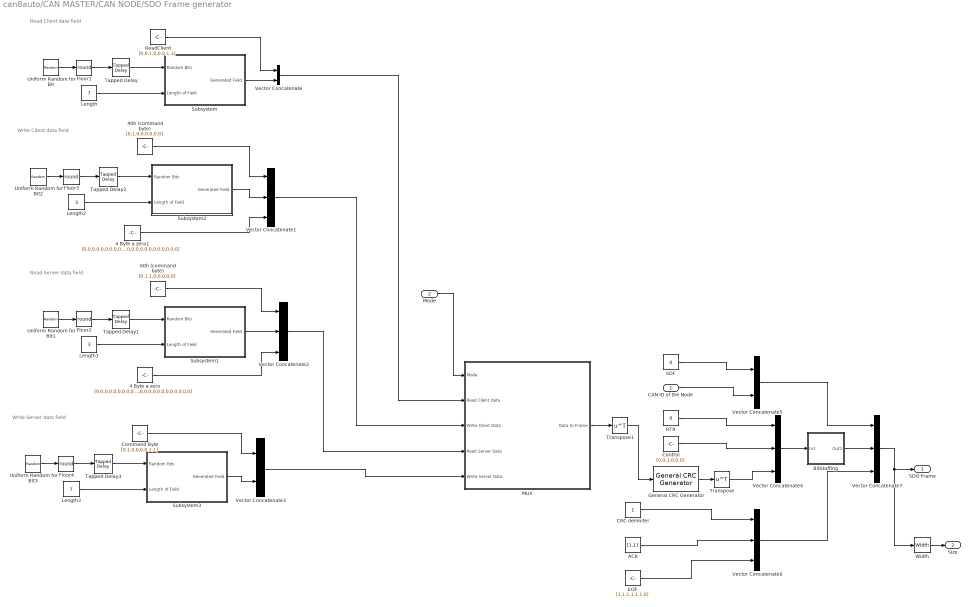
== system can8auto/CAN MASTER/CAN NODE/SDO Frame generator ==
  note: Read Server data field
  note: Read Client data field
  note: Write Client data field
  note: Write Server data field
  CAN ID of the Node : Inport
  Mode : Inport  Port=2
  4 Byte a zero : Constant  Value=[0,0,0,0,0,0,0,0,0,0,0,0,0,0,0,0,0,0,0,0,0,0,0,0,0,0,0,0,0,0,0,0]  VectorParams1D=off
  4 Byte a zero1 : Constant  Value=[0,0,0,0,0,0,0,0,0,0,0,0,0,0,0,0,0,0,0,0,0,0,0,0,0,0,0,0,0,0,0,0]  VectorParams1D=off
  40h (command byte) : Constant  Value=[0,1,0,0,0,0,0,0]  VectorParams1D=off
  60h (command byte) : Constant  Value=[0,1,1,0,0,0,0,0]  VectorParams1D=off
  ACK : Constant  Value=[1,1]  VectorParams1D=off
  BitStuffing : Subsystem
  CRC delimiter : Constant  VectorParams1D=off
  Command Byte : Constant  Value=[0,1,0,0,0,0,1,1]  VectorParams1D=off
  Control : Constant  Value=[0,0,1,0,0,0]  VectorParams1D=off
  EOF : Constant  Value=[1,1,1,1,1,1,0]  VectorParams1D=off
  Floor{1..4} (4 alike) : Rounding  Operator=round
  General CRC Generator : commcrc2/General CRC Generator  genPoly='z^15 + z^14 + z^10 + z^8 + z^7 + z^4 + z^3 + 1'  iniStates=0  directMethod=off  reflectInputBytes=off  reflectChecksums=off  finalXOR=0  numChecksums=1
      settings: SourceProductName=Communications Toolbox  SourceProductBaseCode=CM
  Length : Constant  Value=7  VectorParams1D=off
  Length1 : Constant  Value=3  VectorParams1D=off
  Length2 : Constant  Value=3  VectorParams1D=off
  Length3 : Constant  Value=7  VectorParams1D=off
  MUX : Subsystem
  RTR : Constant  Value=0  VectorParams1D=off
  ReadClient : Constant  Value=[0,0,1,0,0,0,1,1]  VectorParams1D=off
  SOF : Constant  Value=0  VectorParams1D=off
  Subsystem : Subsystem
  Subsystem1 : Subsystem
  Subsystem2 : Subsystem
  Subsystem3 : Subsystem
  Tapped Delay{,1..3} (4 alike) : simulink/Discrete/Tapped Delay  vinit=0  samptime=-1  NumDelays=8*8  DelayOrder=Oldest  includeCurrent=off
  Transpose : Math  Operator=transpose  SaturateOnIntegerOverflow=on
  Transpose1 : Math  Operator=transpose  SaturateOnIntegerOverflow=on
  Uniform Random for Bit{,1..3} (4 alike) : UniformRandomNumber  Minimum=0  SampleTime=0.01
  Vector Concatenate : Concatenate
  Vector Concatenate{1..2,4,6..7} (5 alike) : Concatenate  NumInputs=3
  Vector Concatenate3 : Concatenate
  Vector Concatenate5 : Concatenate
  Width : Width
  SDO Frame : Outport
  " Size" : Outport  Port=2
  wires:
  Vector Concatenate7/1 -> SDO Frame/1, Width/1
  Vector Concatenate5/1 -> Vector Concatenate7/1
  Vector Concatenate6/1 -> Vector Concatenate7/3
  BitStuffing/1(Out1) -> Vector Concatenate7/2
  Vector Concatenate4/1 -> BitStuffing/1(In1)
  RTR/1 -> Vector Concatenate4/1
  CRC delimiter/1 -> Vector Concatenate6/1
  ACK/1 -> Vector Concatenate6/2
  EOF/1 -> Vector Concatenate6/3
  CAN ID of the Node/1 -> Vector Concatenate5/2
  SOF/1 -> Vector Concatenate5/1
  MUX/1(Data to Frame) -> Transpose1/1
  Vector Concatenate3/1 -> MUX/5(Write Server Data)
  Vector Concatenate2/1 -> MUX/4(Read Server Data)
  Mode/1 -> MUX/1(Mode)
  Vector Concatenate1/1 -> MUX/3(Write Client Data)
  Vector Concatenate/1 -> MUX/2(Read Client Data)
  Width/1 -> " Size"/1
  ReadClient/1 -> Vector Concatenate/1
  Floor2/1 -> Tapped Delay1/1
  Subsystem/1(Generated Field) -> Vector Concatenate/2
  General CRC Generator/1 -> Transpose/1
  Length3/1 -> Subsystem3/2(Length of Field)
  Transpose/1 -> Vector Concatenate4/3
  4 Byte a zero/1 -> Vector Concatenate2/3
  4 Byte a zero1/1 -> Vector Concatenate1/3
  Control/1 -> Vector Concatenate4/2
  Subsystem2/1(Generated Field) -> Vector Concatenate1/2
  Tapped Delay1/1 -> Subsystem1/1(Random Bits)
  Floor1/1 -> Tapped Delay/1
  Uniform Random for Bit2/1 -> Floor3/1
  Subsystem1/1(Generated Field) -> Vector Concatenate2/2
  Subsystem3/1(Generated Field) -> Vector Concatenate3/2
  Command Byte/1 -> Vector Concatenate3/1
  Tapped Delay3/1 -> Subsystem3/1(Random Bits)
  Floor4/1 -> Tapped Delay3/1
  40h (command byte)/1 -> Vector Concatenate1/1
  Length2/1 -> Subsystem2/2(Length of Field)
  Uniform Random for Bit1/1 -> Floor2/1
  Length/1 -> Subsystem/2(Length of Field)
  Uniform Random for Bit3/1 -> Floor4/1
  Length1/1 -> Subsystem1/2(Length of Field)
  Tapped Delay/1 -> Subsystem/1(Random Bits)
  Floor3/1 -> Tapped Delay2/1
  Uniform Random for Bit/1 -> Floor1/1
  60h (command byte)/1 -> Vector Concatenate2/1
  Transpose1/1 -> General CRC Generator/1
  Tapped Delay2/1 -> Subsystem2/1(Random Bits)

== system can8auto/CAN MASTER/CAN NODE/SYNC Frame Generator ==
  ACK : Constant  Value=[1,1]  VectorParams1D=off
  BitStuffing : Subsystem
  COB ID (080h) : Constant  Value=[0,0,0,1,0,0,0,0,0,0,0]  VectorParams1D=off
  CRC delimiter : Constant  VectorParams1D=off
  Control : Constant  Value=[0,0,0,0,0,1]  VectorParams1D=off
  Data : Constant  Value=[0,0,0,0,0,0,0,0]'  VectorParams1D=off
  EOF : Constant  Value=[1,1,1,1,1,1,0]  VectorParams1D=off
  General CRC Generator : commcrc2/General CRC Generator  genPoly='z^15 + z^14 + z^10 + z^8 + z^7 + z^4 + z^3 + 1'  iniStates=0  directMethod=off  reflectInputBytes=off  reflectChecksums=off  finalXOR=0  numChecksums=1
      settings: SourceProductName=Communications Toolbox  SourceProductBaseCode=CM
  Mux1 : Mux  Inputs=3
  Mux2 : Mux  Inputs=2
  Mux3 : Mux  Inputs=3
  Mux4 : Mux  Inputs=3
  RTR : Constant  Value=0  VectorParams1D=off
  SOF : Constant  Value=0  VectorParams1D=off
  Transpose : Math  Operator=transpose  SaturateOnIntegerOverflow=on
  Width : Width
  SYNC Frame : Outport
  " Size" : Outport  Port=2
  wires:
  Mux4/1 -> SYNC Frame/1, Width/1
  Mux1/1 -> Mux4/1
  Mux2/1 -> Mux4/3
  BitStuffing/1(Out1) -> Mux4/2
  Mux3/1 -> BitStuffing/1(In1)
  Width/1 -> " Size"/1
  CRC delimiter/1 -> Mux3/3
  EOF/1 -> Mux2/2
  ACK/1 -> Mux2/1
  COB ID (080h)/1 -> Mux1/2
  SOF/1 -> Mux1/1
  Control/1 -> Mux3/1
  General CRC Generator/1 -> Transpose/1
  Transpose/1 -> Mux3/2
  RTR/1 -> Mux1/3
  Data/1 -> General CRC Generator/1

== system can8auto/CAN MASTER/CAN NODE/Triggered Subsystem1 ==
  In1 : Inport
  Trigger : TriggerPort  VariantControl=Variant
  Out1 : Outport  InitialOutput=[1]
  wires:
  In1/1 -> Out1/1

== system can8auto/PDO NODO CAN /CAN NODE/Bootup Frame generator ==
  note: CAN ID / COB ID
  ID of the Node : Inport
  11-bit Adder : Subsystem
  700h : Constant  Value=[1,1,1,0,0,0,0,0,0,0,0]  VectorParams1D=off
  ACK : Constant  Value=[1,1]  VectorParams1D=off
  BitStuffing : Subsystem
  CRC delimiter : Constant  VectorParams1D=off
  Control : Constant  Value=[0,0,0,0,0,1]  VectorParams1D=off
  "Data (Bootup State) " : Constant  Value=[0,0,0,0,0,0,0,0]'  VectorParams1D=off
  EOF : Constant  Value=[1,1,1,1,1,1,0]  VectorParams1D=off
  General CRC Generator : commcrc2/General CRC Generator  genPoly='z^15 + z^14 + z^10 + z^8 + z^7 + z^4 + z^3 + 1'  iniStates=0  directMethod=off  reflectInputBytes=off  reflectChecksums=off  finalXOR=0  numChecksums=1
      settings: SourceProductName=Communications Toolbox  SourceProductBaseCode=CM
  Mux : Mux  Inputs=3
  Mux1 : Mux  Inputs=2
  Mux2 : Mux  Inputs=3
  Mux3 : Mux  Inputs=3
  RTR : Constant  Value=0  VectorParams1D=off
  SOF : Constant  Value=0  VectorParams1D=off
  Transpose : Math  Operator=transpose  SaturateOnIntegerOverflow=on
  Width : Width
  Bootload Frame : Outport
  " Size" : Outport  Port=2
  wires:
  Mux1/1 -> Mux3/1
  Mux2/1 -> Mux3/3
  BitStuffing/1(Out1) -> Mux3/2
  Mux3/1 -> Bootload Frame/1, Width/1
  Transpose/1 -> Mux/3
  RTR/1 -> Mux/1
  EOF/1 -> Mux2/3
  ACK/1 -> Mux2/2
  CRC delimiter/1 -> Mux2/1
  SOF/1 -> Mux1/1
  11-bit Adder/1(Out1) -> Mux1/2
  Width/1 -> " Size"/1
  ID of the Node/1 -> 11-bit Adder/2(In2)
  700h/1 -> 11-bit Adder/1(In1)
  Control/1 -> Mux/2
  "Data (Bootup State) "/1 -> General CRC Generator/1
  General CRC Generator/1 -> Transpose/1
  Mux/1 -> BitStuffing/1(In1)

== system can8auto/PDO NODO CAN /CAN NODE/Frame MUX ==
  Frame Kind : Inport
  Bootload Frame : Inport  Port=2
  Size Bootload : Inport  Port=3
  NMT Frame : Inport  Port=4
  Size NMT : Inport  Port=5
  SDO Frame : Inport  Port=6
  Size SDO : Inport  Port=7
  PDO Frame : Inport  Port=8
  Size PDO : Inport  Port=9
  SYNC Frame : Inport  Port=10
  Size SYNC : Inport  Port=11
  MATLAB Function2 : MATLAB Function  TreatAsAtomicUnit=on
  Vector Concatenate : Concatenate  NumInputs=5
  Vector Concatenate1 : Concatenate  NumInputs=5
  Frame to Send : Outport
  wires:
  Vector Concatenate1/1 -> MATLAB Function2/3(size)
  SYNC Frame/1 -> Vector Concatenate/5
  Size NMT/1 -> Vector Concatenate1/2
  Size SDO/1 -> Vector Concatenate1/3
  Size Bootload/1 -> Vector Concatenate1/1
  Size SYNC/1 -> Vector Concatenate1/5
  Vector Concatenate/1 -> MATLAB Function2/2(u1)
  SDO Frame/1 -> Vector Concatenate/3
  MATLAB Function2/1(result) -> Frame to Send/1
  Bootload Frame/1 -> Vector Concatenate/1
  PDO Frame/1 -> Vector Concatenate/4
  Frame Kind/1 -> MATLAB Function2/1(mode)
  NMT Frame/1 -> Vector Concatenate/2
  Size PDO/1 -> Vector Concatenate1/4

== system can8auto/PDO NODO CAN /CAN NODE/NMT Frame generator ==
  note: DATA FIELD
  Address node : Inport
  11-bit Adder : Subsystem
  ACK : Constant  Value=[1,1]  VectorParams1D=off
  BitStuffing : Subsystem
  COB ID : Constant  Value=[0,0,0,0,0,0,0,0,0,0,0]  VectorParams1D=off
  CRC delimiter : Constant  VectorParams1D=off
  Control : Constant  Value=[0,0,0,0,1,0]  VectorParams1D=off
  DATA (part1) : Constant  Value=[0,0,0,0,0]  VectorParams1D=off
  "Data " : Constant  Value=[0,0,1,0,0,0,0,0,0,0,0]  VectorParams1D=off
  EOF : Constant  Value=[1,1,1,1,1,1,0]  VectorParams1D=off
  General CRC Generator : commcrc2/General CRC Generator  genPoly='z^15 + z^14 + z^10 + z^8 + z^7 + z^4 + z^3 + 1'  iniStates=0  directMethod=off  reflectInputBytes=off  reflectChecksums=off  finalXOR=0  numChecksums=1
      settings: SourceProductName=Communications Toolbox  SourceProductBaseCode=CM
  Mux : Mux  Inputs=3
  Mux1 : Mux  Inputs=2
  Mux2 : Mux  Inputs=2
  Mux3 : Mux  Inputs=3
  Mux4 : Mux  Inputs=3
  RTR : Constant  Value=0  VectorParams1D=off
  SOF : Constant  Value=0  VectorParams1D=off
  Transpose : Math  Operator=transpose  SaturateOnIntegerOverflow=on
  Transpose1 : Math  Operator=transpose  SaturateOnIntegerOverflow=on
  Width : Width
  NMT Frame : Outport
  " Size" : Outport  Port=2
  wires:
  Mux4/1 -> Width/1, NMT Frame/1
  Mux3/1 -> Mux4/3
  Mux2/1 -> Mux4/1
  BitStuffing/1(Out1) -> Mux4/2
  Mux/1 -> BitStuffing/1(In1)
  RTR/1 -> Mux/1
  CRC delimiter/1 -> Mux3/1
  ACK/1 -> Mux3/2
  EOF/1 -> Mux3/3
  SOF/1 -> Mux2/1
  COB ID/1 -> Mux2/2
  Width/1 -> " Size"/1
  Transpose1/1 -> General CRC Generator/1
  Mux1/1 -> Transpose1/1
  11-bit Adder/1(Out1) -> Mux1/2
  DATA (part1)/1 -> Mux1/1
  "Data "/1 -> 11-bit Adder/1(In1)
  Address node/1 -> 11-bit Adder/2(In2)
  Transpose/1 -> Mux/3
  Control/1 -> Mux/2
  General CRC Generator/1 -> Transpose/1

== system can8auto/PDO NODO CAN /CAN NODE/PDO Frame Generator ==
  note: PDO DATA field
  note: CONTROL field
  CAN ID : Inport
  Data Length : Inport  Port=2
  " default = 8" : SwitchCase  CaseConditions={2,4}
  2 byte : Constant  Value=[0,0,0,0,1,0]  VectorParams1D=off
  4 byte : Constant  Value=[0,0,0,1,0,0]  VectorParams1D=off
  8 byte : Constant  Value=[0,0,1,0,0,0]  VectorParams1D=off
  ACK : Constant  Value=[1,1]  VectorParams1D=off
  CRC delimiter : Constant  VectorParams1D=off
  EOF : Constant  Value=[1,1,1,1,1,1,0]  VectorParams1D=off
  Floor1 : Rounding  Operator=round
  General CRC Generator : commcrc2/General CRC Generator  genPoly='z^15 + z^14 + z^10 + z^8 + z^7 + z^4 + z^3 + 1'  iniStates=0  directMethod=off  reflectInputBytes=off  reflectChecksums=off  finalXOR=0  numChecksums=1
      settings: SourceProductName=Communications Toolbox  SourceProductBaseCode=CM
  Merge1 : Merge  Inputs=3
  RTR : Constant  Value=0  VectorParams1D=off
  SOF : Constant  Value=0  VectorParams1D=off
  Subsystem : Subsystem
  Switch Case Action Subsystem : Subsystem  TreatAsAtomicUnit=on
  Switch Case Action Subsystem1 : Subsystem  TreatAsAtomicUnit=on
  Switch Case Action Subsystem2 : Subsystem  TreatAsAtomicUnit=on
  Tapped Delay : simulink/Discrete/Tapped Delay  vinit=0  samptime=-1  NumDelays=8*8  DelayOrder=Oldest  includeCurrent=off
  Uniform Random for Bit : UniformRandomNumber  Minimum=0  SampleTime=0.01
  Vector Concatenate1 : Concatenate  NumInputs=8
  Width : Width
  PDO Frame : Outport
  " Size" : Outport  Port=2
  wires:
  Vector Concatenate1/1 -> PDO Frame/1, Width/1
  Width/1 -> " Size"/1
  ACK/1 -> Vector Concatenate1/7
  EOF/1 -> Vector Concatenate1/8
  General CRC Generator/1 -> Vector Concatenate1/5
  Switch Case Action Subsystem1/1(Out1) -> Merge1/2
  2 byte/1 -> Switch Case Action Subsystem/1(In1)
  Tapped Delay/1 -> Subsystem/1(Random Bits)
  RTR/1 -> Vector Concatenate1/3
  Uniform Random for Bit/1 -> Floor1/1
  " default = 8"/3 -> Switch Case Action Subsystem2/Action
  Floor1/1 -> Tapped Delay/1
  SOF/1 -> Vector Concatenate1/1
  Data Length/1 -> " default = 8"/1, Subsystem/2(Length of Field)
  4 byte/1 -> Switch Case Action Subsystem1/1(In1)
  Subsystem/1(Generated Field) -> General CRC Generator/1
  " default = 8"/1 -> Switch Case Action Subsystem/Action
  CRC delimiter/1 -> Vector Concatenate1/6
  Merge1/1 -> Vector Concatenate1/4
  " default = 8"/2 -> Switch Case Action Subsystem1/Action
  8 byte/1 -> Switch Case Action Subsystem2/1(In1)
  CAN ID/1 -> Vector Concatenate1/2
  Switch Case Action Subsystem2/1(Out1) -> Merge1/3
  Switch Case Action Subsystem/1(Out1) -> Merge1/1
